simulink model "sampleModel63"  (R2021b)
settings: Solver=VariableStepAuto  StartTime=0.0  StopTime=10.0  RelTol=1e-3
undefined symbols (not defined in the file or in its folder): DiscIntNeverNeededParam, Newton, Raphson
libraries: simulink x12, slpidlib x2
settings Model: Creator=user  LastModifiedBy=user

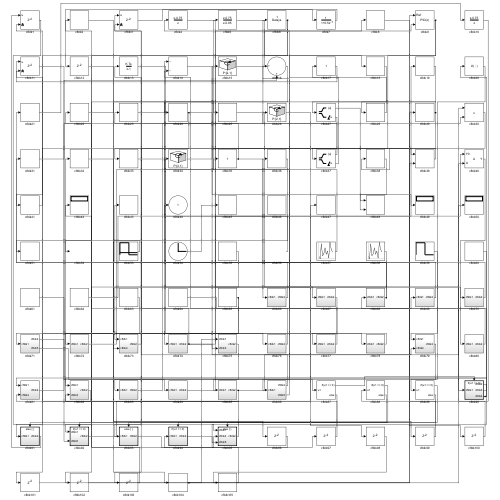
[thumbnail: Simulink's stored preview of the top-level diagram]
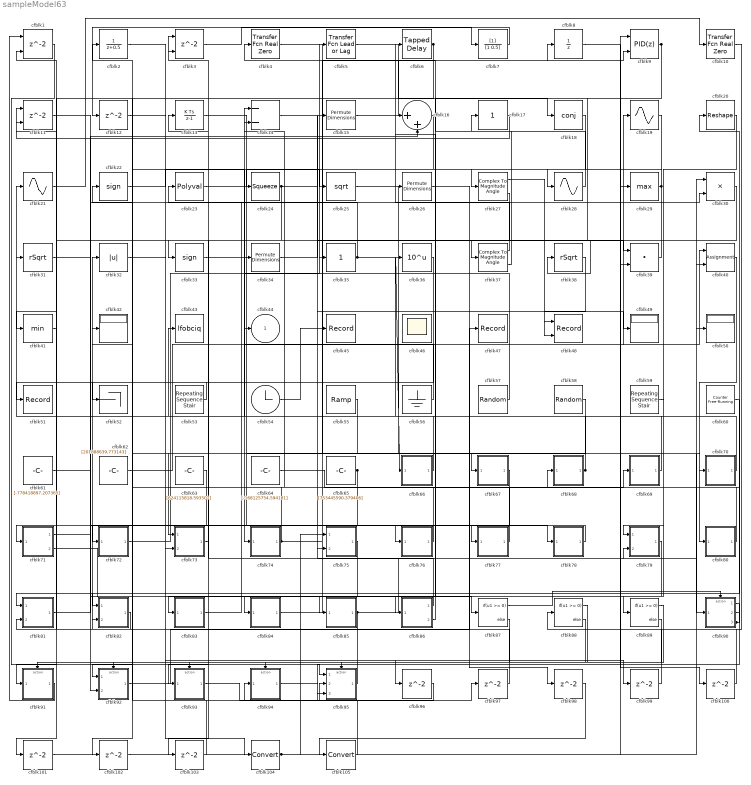
== system sampleModel63 ==
  cfblk1 : Delay  ShowEnablePort=on  SampleTime=1
      settings: InputPortMap=u0,e6
  cfblk10 : simulink/Discrete/Transfer Fcn Real Zero  ZeroZ=0.75  ICPrevInput=0.0  DoSatur=off
      settings: SourceProductBaseCode=SL
  cfblk{12,96..103} (9 alike) : Delay  SampleTime=1
  cfblk104 : DataTypeConversion
  cfblk105 : DataTypeConversion
  cfblk11 : Delay  ShowEnablePort=on  SampleTime=1
      settings: InputPortMap=u0,e6
  cfblk13 : DiscreteIntegrator  ICPrevOutput=DiscIntNeverNeededParam  ICPrevScaledInput=DiscIntNeverNeededParam
  cfblk14 : Sum  Inputs=--
  cfblk15 : PermuteDimensions
  cfblk16 : Sum  Inputs=|++
  cfblk17 : simulink/Math Operations/Slider Gain  gain=1  low=0  high=2
  cfblk18 : Math  Operator=conj  SaturateOnIntegerOverflow=on
  cfblk19 : Sin  TimeSource=Use external signal  SampleTime=0
  cfblk2 : DiscreteTransferFcn  SampleTime=1
  cfblk20 : Reshape
  cfblk21 : Sin  TimeSource=Use external signal  SampleTime=0
  cfblk22 : Signum
  cfblk23 : Polyval  Coefs=[ +2.081618890e-019, -1.441693666e-014, +4.719686976e-010, -8.536869453e-006, +1.621573104e-001, -8.087801117e+001 ]
  cfblk24 : Squeeze
  cfblk25 : Sqrt  SaturateOnIntegerOverflow=on
  cfblk26 : PermuteDimensions
  cfblk27 : ComplexToMagnitudeAngle
  cfblk28 : Sin  TimeSource=Use external signal  SampleTime=0
  cfblk29 : MinMax  Function=max
  cfblk3 : Delay  ShowEnablePort=on  SampleTime=1
      settings: InputPortMap=u0,e6
  cfblk30 : Product  Inputs=**
  cfblk31 : Sqrt  Operator=rSqrt  AlgorithmType=Newton-Raphson  SaturateOnIntegerOverflow=on
  cfblk32 : Abs
  cfblk33 : Signum
  cfblk34 : PermuteDimensions
  cfblk35 : simulink/Math Operations/Slider Gain  gain=1  low=0  high=2
  cfblk36 : Math  Operator=10^u  SaturateOnIntegerOverflow=on
  cfblk37 : ComplexToMagnitudeAngle
  cfblk38 : Sqrt  Operator=rSqrt  AlgorithmType=Newton-Raphson  SaturateOnIntegerOverflow=on
  cfblk39 : DotProduct  InputSameDT=on  OutDataTypeStr=Inherit: Inherit via internal rule
  cfblk4 : simulink/Discrete/Transfer Fcn Real Zero  ZeroZ=0.75  ICPrevInput=0.0  DoSatur=off
      settings: SourceProductBaseCode=SL
  cfblk40 : Assignment  DiagnosticForDimensions=Warning  IndexOptions=Index vector (dialog)  Indices=1  OutputSizes=1
  cfblk41 : MinMax
  cfblk42 : Display
  cfblk43 : ToWorkspace  VariableName=lfobciq  SaveFormat=Timeseries  SampleTime=-1
  cfblk45 : Record  FileSettingsInternal="{\"entries\":[{\"content\":{\"excelSettings\":{\"content\":{},\"type\":\"Streamout.ExcelSettings\"}},\"type\":\"Streamout.FileSettingStorage\",\"uuid\":\"eab00038-920a-4507-b0a5-0f8dc5558c4e\"}],\"packageUris\":[\"http://schema.mathworks.com/mf0/streamout_blocks/R2020a\"],\"version\":\"1.0\"}"  SignalsInternal="{\"entries\":[{\"content\":{\"signals\":[{\"content\":{\"blockPath\":[\"sampleModel63/cfblk45\"],\"channel\":[],\"dimensions\":[1],\"domain\":\"sampleModel63/cfblk45\",\"lineColor\":\"#7e2f8e\",\"plots\":[1],\"port\":1,\"sid\":[\"\"],\"signalID\":2453,\"signalName\":\"cfblk54\"},\"type\":\"RecordBlkView.Signal\",\"uuid\":\"6f20d37a-a5dd-4b7e-9677-872bf411aa66\"}]},\"type\":\"RecordBlkView.InputSignals\",\"uuid\":\"9bafe70f-6cc7-4dfb-b2fd-3a91eeb87f2c\"}],\"packageUris\":[\"http://schema.mathworks.com/mf0/streamout_blocks/R2020a\"],\"version\":\"1.0\"}"  VisualizationBindings="{\"sparklinesplugin\":{\"info\":[{\"bindingParametersList\":[],\"subplotID\":1}]}}"
  cfblk46 : Scope
      settings: Floating=on
  cfblk47 : Record  FileSettingsInternal="{\"entries\":[{\"content\":{\"excelSettings\":{\"content\":{},\"type\":\"Streamout.ExcelSettings\"}},\"type\":\"Streamout.FileSettingStorage\",\"uuid\":\"8624b493-b75b-4048-a20b-65c7ffb17f01\"}],\"packageUris\":[\"http://schema.mathworks.com/mf0/streamout_blocks/R2020a\"],\"version\":\"1.0\"}"  SignalsInternal="{\"entries\":[{\"content\":{\"signals\":[{\"content\":{\"blockPath\":[\"sampleModel63/cfblk47\"],\"channel\":[],\"dimensions\":[1],\"domain\":\"sampleModel63/cfblk47\",\"lineColor\":\"#0072bd\",\"plots\":[1],\"port\":1,\"sid\":[\"\"],\"signalID\":2441,\"signalName\":\"cfblk92\"},\"type\":\"RecordBlkView.Signal\",\"uuid\":\"a7be9c3a-7afb-4874-9450-2f20fa88f380\"}]},\"type\":\"RecordBlkView.InputSignals\",\"uuid\":\"be4317a2-c2d3-43f3-bc84-726c03d485cb\"}],\"packageUris\":[\"http://schema.mathworks.com/mf0/streamout_blocks/R2020a\"],\"version\":\"1.0\"}"  VisualizationBindings="{\"sparklinesplugin\":{\"info\":[{\"bindingParametersList\":[],\"subplotID\":1}]}}"
  cfblk48 : Record  FileSettingsInternal="{\"entries\":[{\"content\":{\"excelSettings\":{\"content\":{},\"type\":\"Streamout.ExcelSettings\"}},\"type\":\"Streamout.FileSettingStorage\",\"uuid\":\"a40df8e6-25e3-4f39-8082-43196c5c9d58\"}],\"packageUris\":[\"http://schema.mathworks.com/mf0/streamout_blocks/R2020a\"],\"version\":\"1.0\"}"  Layout=[1 1]  SignalsInternal="{\"entries\":[{\"content\":{\"signals\":[{\"content\":{\"blockPath\":[\"sampleModel63/cfblk48\"],\"channel\":[],\"dimensions\":[1,1],\"domain\":\"sampleModel63/cfblk48\",\"lineColor\":\"#a2142f\",\"plots\":[1],\"port\":1,\"sid\":[\"\"],\"signalID\":2445,\"signalName\":\"cfblk27:1\"},\"type\":\"RecordBlkView.Signal\",\"uuid\":\"b3ce3bcc-e12a-4239-8f85-80006c98ae86\"},{\"content\":{\"blockPath\":[\"sampleModel63/cfblk48\"],\"channel\":[],\"dimensions\":[1,1],\"domain\":\"sampleModel63/cfblk48\",\"lineColor\":\"#139fff\",\"plots\":[1],\"port\":2,\"sid\":[\"\"],\"signalID\":2449,\"signalName\":\"cfblk38\"},\"type\":\"RecordBlkView.Signal\",\"uuid\":\"d8960520-a3b1-4adb-9b58-2e04172c18e8\"}]},\"type\":\"RecordBlkView.InputSignals\",\"uuid\":\"834f0da8-eec6-4e4f-9565-3c19297e5a2d\"}],\"packageUris\":[\"http://schema.mathworks.com/mf0/streamout_blocks/R2020a\"],\"version\":\"1.0\"}"  VisualizationBindings="{\"xyplotplugin\":{\"info\":[{\"series\":[{\"bindingParametersList\":[{\"parameter\":\"X-Axis\",\"signalID\":2445,\"signalName\":\"cfblk27:1\"},{\"parameter\":\"Y-Axis\",\"signalID\":2449,\"signalName\":\"cfblk38\"}],\"seriesID\":5141}],\"subplotID\":1}]}}"  CompatibilityTag=XY
  cfblk49 : Display
  cfblk5 : simulink/Discrete/Transfer Fcn Lead or Lag  PoleZ=0.95  ZeroZ=0.75  ICPrevOutput=0.0  ICPrevInput=0.0  DoSatur=off
      settings: SourceProductBaseCode=SL
  cfblk50 : Display
  cfblk51 : Record  FileSettingsInternal="{\"entries\":[{\"content\":{\"excelSettings\":{\"content\":{},\"type\":\"Streamout.ExcelSettings\"}},\"type\":\"Streamout.FileSettingStorage\",\"uuid\":\"85545bd8-52c1-4d99-9c40-672c6dfcf42a\"}],\"packageUris\":[\"http://schema.mathworks.com/mf0/streamout_blocks/R2020a\"],\"version\":\"1.0\"}"  SignalsInternal="{\"entries\":[{\"content\":{\"signals\":[{\"content\":{\"blockPath\":[\"sampleModel63/cfblk51\"],\"channel\":[],\"dimensions\":[1],\"domain\":\"sampleModel63/cfblk51\",\"lineColor\":\"#77ac30\",\"plots\":[1],\"port\":1,\"sid\":[\"\"],\"signalID\":2457,\"signalName\":\"cfblk53\"},\"type\":\"RecordBlkView.Signal\",\"uuid\":\"2fbab494-daff-4625-9a56-065129460eaf\"}]},\"type\":\"RecordBlkView.InputSignals\",\"uuid\":\"dac925e5-03f2-4dde-8f24-8a4a20c8e071\"}],\"packageUris\":[\"http://schema.mathworks.com/mf0/streamout_blocks/R2020a\"],\"version\":\"1.0\"}"  VisualizationBindings="{\"sparklinesplugin\":{\"info\":[{\"bindingParametersList\":[],\"subplotID\":1}]}}"
  cfblk52 : Terminator
  cfblk53 : simulink/Sources/Repeating Sequence Stair  OutValues=[503450450.521379, -107905093.515396]  tsamp=-1  OutMin=[]  OutMax=[]  OutDataTypeStr=double  OutputDataTypeScalingMode=double  OutDataType=fixdt(0,8)  ConRadixGroup=Best Precision: Vector-wise  OutScaling=2^-12
  cfblk54 : Clock
  cfblk55 : simulink/Sources/Ramp  slope=[-5371.335129]  start=[28.819203]  InitialOutput=[-574228.703144]
  cfblk56 : Ground
  cfblk57 : UniformRandomNumber  Minimum=[-7281642111.005922]  Maximum=[1759054305.272253]  Seed=[77560895.000000]  SampleTime=0.1
  cfblk58 : UniformRandomNumber  Minimum=[-9181369548.878405]  Maximum=[5487264494.618241]  Seed=[73205660.000000]  SampleTime=0.1
  cfblk59 : simulink/Sources/Repeating Sequence Stair  OutValues=[306494964.090970, 306068425.132044]  tsamp=-1  OutMin=[]  OutMax=[]  OutDataTypeStr=double  OutputDataTypeScalingMode=double  OutDataType=fixdt(0,8)  ConRadixGroup=Best Precision: Vector-wise  OutScaling=2^-12
  cfblk6 : simulink/Discrete/Tapped Delay  vinit=0.0  samptime=-1  NumDelays=1  DelayOrder=Oldest  includeCurrent=off
  cfblk60 : simulink/Sources/Counter Free-Running  NumBits=[41.000000]  tsamp=-1
  cfblk61 : Constant  Value=[-778418897.207365]  SampleTime=1
  cfblk62 : Constant  Value=[201888639.773143]  SampleTime=1
  cfblk63 : Constant  Value=[624115818.593507]  SampleTime=1
  cfblk64 : Constant  Value=[-168125754.594181]  SampleTime=1
  cfblk65 : Constant  Value=[753445590.379406]  SampleTime=1
  cfblk66 : Subsystem
  cfblk67 : Subsystem
  cfblk68 : Subsystem
  cfblk69 : Subsystem
  cfblk7 : DiscreteFilter  SampleTime=1
  cfblk70 : Subsystem
  cfblk71 : Subsystem
  cfblk72 : Subsystem
  cfblk73 : Subsystem
  cfblk74 : Subsystem
  cfblk75 : Subsystem
  cfblk76 : Subsystem
  cfblk77 : Subsystem
  cfblk78 : Subsystem
  cfblk79 : Subsystem
  cfblk8 : UnitDelay  HasFrameUpgradeWarning=on
  cfblk80 : Subsystem
  cfblk81 : Subsystem
  cfblk82 : Subsystem
  cfblk83 : Subsystem
  cfblk84 : Subsystem
  cfblk85 : Subsystem
  cfblk86 : Subsystem
  cfblk87 : If  IfExpression=u1 >= 0  SampleTime=1
  cfblk88 : If  IfExpression=u1 >= 0  SampleTime=1
  cfblk89 : If  IfExpression=u1 >= 0  SampleTime=1
  cfblk9 : slpidlib/PID Controller (2DOF)  Controller=PID  Form=Parallel  TimeDomain=Discrete-time  UseExternalTs=off  SampleTime=1  IntegratorMethod=Forward Euler  FilterMethod=Forward Euler  ControllerParametersSource=internal  P=1  I=1  D=0  UseFilter=on  N=100  b=1  c=1  TunerSelectOption=Transfer Function Based (PID Tuner App)  InitialConditionSource=internal  InitialConditionForIntegrator=0  InitialConditionForFilter=0  DifferentiatorICPrevScaledInput=0  ExternalReset=none  TrackingMode=off  Kt=1  LimitOutput=off  SatLimitsSource=internal  UpperSaturationLimit=inf  LowerSaturationLimit=-inf  LinearizeAsGain=off  AntiWindupMode=none  Kb=1  POutMin=[]  POutMax=[]  IOutMin=[]  IOutMax=[]  DOutMin=[]  DOutMax=[]  NOutMin=[]  NOutMax=[]  bOutMin=[]  bOutMax=[]  cOutMin=[]  cOutMax=[]  SumOutMin=[]  SumOutMax=[]  SaturationOutMin=[]  SaturationOutMax=[]  PParamMin=[]  PParamMax=[]  IParamMin=[]  IParamMax=[]  DParamMin=[]  DParamMax=[]  NParamMin=[]  NParamMax=[]  bParamMin=[]  bParamMax=[]  cParamMin=[]  cParamMax=[]  KbParamMin=[]  KbParamMax=[]  KtParamMin=[]  KtParamMax=[]  KbOutMin=[]  KbOutMax=[]  KtOutMin=[]  KtOutMax=[]  IntegratorOutMin=[]  IntegratorOutMax=[]  FilterOutMin=[]  FilterOutMax=[]  SumI1OutMin=[]  SumI1OutMax=[]  SumI2OutMin=[]  SumI2OutMax=[]  SumI3OutMin=[]  SumI3OutMax=[]  SumI4OutMin=[]  SumI4OutMax=[]  SumDOutMin=[]  SumDOutMax=[]  Sum1OutMin=[]  Sum1OutMax=[]  Sum2OutMin=[]  Sum2OutMax=[]  Sum3OutMin=[]  Sum3OutMax=[]  DifferentiatorOutMin=[]  DifferentiatorOutMax=[]  FilterDiffOutCoefMin=[]  FilterDiffOutCoefMax=[]  ReciprocalOutMin=[]  ReciprocalOutMax=[]  SumDenOutMin=[]  SumDenOutMax=[]  SumNumOutMin=[]  SumNumOutMax=[]  DivideOutMin=[]  DivideOutMax=[]  UdiffTsProdOutMin=[]  UdiffTsProdOutMax=[]  NTsProdOutMin=[]  NTsProdOutMax=[]  UintegralTsProdOutMin=[]  UintegralTsProdOutMax=[]  UngainTsProdOutMin=[]  UngainTsProdOutMax=[]  IntegratorContinuousStateAttributes=''  IntegratorStateMustResolveToSignalObject=off  IntegratorRTWStateStorageClass=Auto  FilterContinuousStateAttributes=''  FilterStateMustResolveToSignalObject=off  FilterRTWStateStorageClass=Auto  ParallelPVariant=InternalParameters  IdealPVariant=Disabled  IVariant=InternalParameters  DVariant=InternalParameters  bVariant=InternalParameters  cVariant=InternalParameters  IntegratorVariant=Discrete  SatVariant=Disabled  AWVariant=Passthrough  PCopyVariant=Disabled  TRVariant=Disabled  FdbkBlocksVariant=Forward  IdealPFdbkVariant=Disabled  SatFdbkVariant=Disabled  DerivativeFilterVariant=ForwardEulerFilter  NVariant=InternalParameters  NCopyVariant=Disabled  FilterICVariant=InternalICsFilter  IntegratorICVariant=InternalICs  ExternalResetVariant=Disabled  TRSumVariant=Passthrough  SumFdbkVariant=Disabled  SumVariant=Sum_PID  TsampFilterVariant=InternalTs  TsampNgainVariant=Passthrough  TsampIntegralVariant=Passthrough  ExternalSaturationOutDataTypeStr=Inherit: Same as second input
      settings: SourceProductBaseCode=SL
  cfblk90 : Subsystem  TreatAsAtomicUnit=on
  cfblk91 : Subsystem  TreatAsAtomicUnit=on
  cfblk92 : Subsystem  TreatAsAtomicUnit=on
  cfblk93 : Subsystem  TreatAsAtomicUnit=on
  cfblk94 : Subsystem  TreatAsAtomicUnit=on
  cfblk95 : Subsystem  TreatAsAtomicUnit=on
  cfblk44 : Outport
  wires:
  cfblk28/1 -> cfblk4/1
  cfblk40/1 -> cfblk80/1(cfblk1)
  cfblk24/1 -> cfblk49/1, cfblk103/1
  cfblk60/1 -> cfblk81/1(cfblk1)
  cfblk9/1 -> cfblk33/1, cfblk86/1(cfblk1)
  cfblk1/1 -> cfblk95/1(cfblk1)
  cfblk68/1(cfblk2) -> cfblk21/1, cfblk36/1
  cfblk35/1 -> cfblk66/1(cfblk1), cfblk3/2
  cfblk4/1 -> cfblk67/1(cfblk1)
  cfblk29/1 -> cfblk38/1, cfblk27/1
  cfblk82/1(cfblk2) -> cfblk81/2(cfblk4)
  cfblk25/1 -> cfblk90/1(cfblk1)
  cfblk10/1 -> cfblk88/1
  cfblk70/1(cfblk2) -> cfblk31/1
  cfblk7/1 -> cfblk12/1
  cfblk95/1(cfblk2) -> cfblk32/1
  cfblk27/1 -> cfblk48/1
  cfblk64/1 -> cfblk69/1(cfblk1)
  cfblk20/1 -> cfblk89/1
  cfblk72/1(cfblk2) -> cfblk5/1
  cfblk69/1(cfblk2) -> cfblk14/1
  cfblk3/1 -> cfblk7/1
  cfblk75/1(cfblk2) -> cfblk83/1(cfblk1)
  cfblk21/1 -> cfblk10/1
  cfblk84/1(cfblk2) -> cfblk9/2
  cfblk53/1 -> cfblk51/1
  cfblk18/1 -> cfblk74/1(cfblk1)
  cfblk54/1 -> cfblk45/1
  cfblk62/1 -> cfblk19/1
  cfblk30/1 -> cfblk41/1
  cfblk57/1 -> cfblk35/1
  cfblk11/1 -> cfblk78/1(cfblk1)
  cfblk5/1 -> cfblk18/1
  cfblk78/1(cfblk2) -> cfblk71/1(cfblk1)
  cfblk34/1 -> cfblk15/1
  cfblk19/1 -> cfblk28/1
  cfblk65/1 -> cfblk72/1(cfblk1), cfblk93/1(cfblk1)
  cfblk92/1(cfblk2) -> cfblk47/1
  cfblk73/1(cfblk2) -> cfblk3/1
  cfblk67/1(cfblk2) -> cfblk77/1(cfblk1)
  cfblk93/1(cfblk2) -> cfblk95/2(cfblk4)
  cfblk13/1 -> cfblk76/1(cfblk1)
  cfblk14/1 -> cfblk39/1
  cfblk63/1 -> cfblk91/1(cfblk1)
  cfblk90/1(cfblk2) -> cfblk95/3(cfblk5)
  cfblk6/1 -> cfblk101/1, cfblk102/1
  cfblk16/1 -> cfblk52/1
  cfblk74/1(cfblk2) -> cfblk40/1, cfblk42/1, cfblk79/2(cfblk4)
  cfblk71/1(cfblk2) -> cfblk84/1(cfblk1)
  cfblk37/1 -> cfblk6/1
  cfblk79/1(cfblk2) -> cfblk85/1(cfblk1)
  cfblk66/1(cfblk2) -> cfblk43/1
  cfblk33/1 -> cfblk70/1(cfblk1)
  cfblk37/2 -> cfblk17/1
  cfblk55/1 -> cfblk73/1(cfblk1)
  cfblk41/1 -> cfblk11/1
  cfblk71/2(cfblk5) -> cfblk87/1
  cfblk36/1 -> cfblk73/2(cfblk4)
  cfblk15/1 -> cfblk8/1
  cfblk39/1 -> cfblk37/1
  cfblk2/1 -> cfblk104/1
  cfblk56/1 -> cfblk44/1
  cfblk91/1(cfblk2) -> cfblk1/1
  cfblk77/1(cfblk2) -> cfblk16/1
  cfblk27/2 -> cfblk75/2(cfblk3)
  cfblk90/2(cfblk3) -> cfblk82/1(cfblk1)
  cfblk86/1(cfblk2) -> cfblk23/1
  cfblk23/1 -> cfblk25/1
  cfblk90/3(cfblk4) -> cfblk68/1(cfblk1), cfblk20/1
  cfblk59/1 -> cfblk79/1(cfblk1)
  cfblk76/1(cfblk2) -> cfblk14/2
  cfblk22/1 -> cfblk24/1
  cfblk31/1 -> cfblk16/2
  cfblk81/1(cfblk2) -> cfblk26/1
  cfblk85/1(cfblk2) -> cfblk50/1, cfblk82/2(cfblk3)
  cfblk17/1 -> cfblk11/2
  cfblk80/1(cfblk2) -> cfblk13/1
  cfblk83/1(cfblk2) -> cfblk30/2
  cfblk58/1 -> cfblk92/1(cfblk1)
  cfblk38/1 -> cfblk48/2
  cfblk86/2(cfblk5) -> cfblk34/1
  cfblk61/1 -> cfblk92/2(cfblk5)
  cfblk87/1 -> cfblk90/Action
  cfblk87/2 -> cfblk91/Action
  cfblk88/1 -> cfblk92/Action
  cfblk88/2 -> cfblk93/Action
  cfblk89/1 -> cfblk94/Action
  cfblk89/2 -> cfblk95/Action
  cfblk32/1 -> cfblk96/1
  cfblk96/1 -> cfblk94/1(cfblk1)
  cfblk94/1(cfblk2) -> cfblk97/1
  cfblk97/1 -> cfblk1/2
  cfblk26/1 -> cfblk98/1
  cfblk12/1 -> cfblk99/1
  cfblk99/1 -> cfblk9/1
  cfblk8/1 -> cfblk100/1
  cfblk100/1 -> cfblk30/1
  cfblk101/1 -> cfblk39/2
  cfblk102/1 -> cfblk40/2
  cfblk103/1 -> cfblk22/1
  cfblk104/1 -> cfblk29/1, cfblk75/1(cfblk1)
  cfblk98/1 -> cfblk105/1
  cfblk105/1 -> cfblk2/1

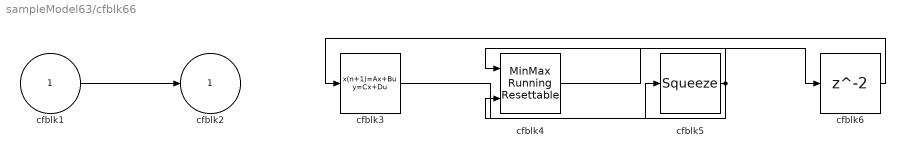
== system sampleModel63/cfblk66 ==
  cfblk1 : Inport
  cfblk3 : DiscreteStateSpace
  cfblk4 : simulink/Math Operations/MinMax Running Resettable  Function=min  vinit=0.0
  cfblk5 : Squeeze
  cfblk6 : Delay  SampleTime=1
  cfblk2 : Outport
  wires:
  cfblk5/1 -> cfblk4/1, cfblk4/2
  cfblk3/1 -> cfblk5/1
  cfblk1/1 -> cfblk2/1
  cfblk4/1 -> cfblk6/1
  cfblk6/1 -> cfblk3/1

== system sampleModel63/cfblk67 ==
  cfblk1 : Inport
  cfblk3 : DiscreteStateSpace
  cfblk2 : Outport
  wires:
  cfblk1/1 -> cfblk2/1, cfblk3/1

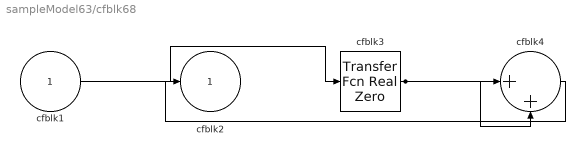
== system sampleModel63/cfblk68 ==
  cfblk1 : Inport
  cfblk3 : simulink/Discrete/Transfer Fcn Real Zero  ZeroZ=0.75  ICPrevInput=0.0  DoSatur=off
      settings: SourceProductBaseCode=SL
  cfblk4 : Sum  Inputs=|++
  cfblk2 : Outport
  wires:
  cfblk1/1 -> cfblk3/1
  cfblk4/1 -> cfblk2/1
  cfblk3/1 -> cfblk4/1, cfblk4/2

== system sampleModel63/cfblk69 ==
  cfblk1 : Inport
  cfblk3 : Sum  Inputs=+
  cfblk2 : Outport
  wires:
  cfblk1/1 -> cfblk3/1
  cfblk3/1 -> cfblk2/1

== system sampleModel63/cfblk70 ==
  cfblk1 : Inport
  cfblk3 : Constant  Value=[-469979118.502152]  SampleTime=1
  cfblk2 : Outport
  wires:
  cfblk1/1 -> cfblk2/1

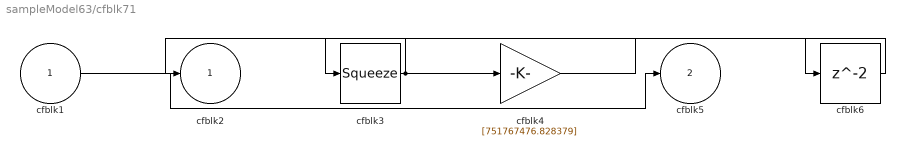
== system sampleModel63/cfblk71 ==
  cfblk1 : Inport
  cfblk3 : Squeeze
  cfblk4 : Gain  Gain=[751767476.828379]
  cfblk6 : Delay  SampleTime=1
  cfblk2 : Outport
  cfblk5 : Outport  Port=2
  wires:
  cfblk1/1 -> cfblk5/1
  cfblk3/1 -> cfblk2/1, cfblk4/1
  cfblk4/1 -> cfblk6/1
  cfblk6/1 -> cfblk3/1

== system sampleModel63/cfblk72 ==
  cfblk1 : Inport
  cfblk3 : Sin  TimeSource=Use external signal  SampleTime=0
  cfblk2 : Outport
  wires:
  cfblk1/1 -> cfblk3/1
  cfblk3/1 -> cfblk2/1

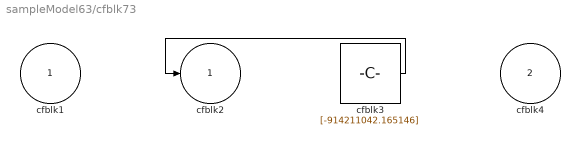
== system sampleModel63/cfblk73 ==
  cfblk1 : Inport
  cfblk4 : Inport  Port=2
  cfblk3 : Constant  Value=[-914211042.165146]  SampleTime=1
  cfblk2 : Outport
  wires:
  cfblk3/1 -> cfblk2/1

== system sampleModel63/cfblk74 ==
  cfblk1 : Inport
  cfblk3 : Bias  Bias=[-714518789.480261]
  cfblk2 : Outport
  wires:
  cfblk3/1 -> cfblk2/1
  cfblk1/1 -> cfblk3/1

== system sampleModel63/cfblk75 ==
  cfblk1 : Inport
  cfblk3 : Inport  Port=2
  cfblk2 : Outport
  wires:
  cfblk3/1 -> cfblk2/1

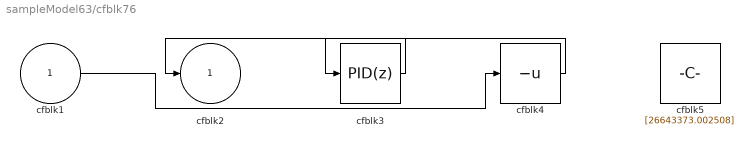
== system sampleModel63/cfblk76 ==
  cfblk1 : Inport
  cfblk3 : slpidlib/PID Controller  Controller=PID  Form=Parallel  TimeDomain=Discrete-time  UseExternalTs=off  SampleTime=1  IntegratorMethod=Forward Euler  FilterMethod=Forward Euler  ControllerParametersSource=internal  P=1  I=1  D=0  UseFilter=on  N=100  TunerSelectOption=Transfer Function Based (PID Tuner App)  InitialConditionSource=internal  InitialConditionForIntegrator=0  InitialConditionForFilter=0  DifferentiatorICPrevScaledInput=0  ExternalReset=none  TrackingMode=off  Kt=1  LimitOutput=off  SatLimitsSource=internal  UpperSaturationLimit=inf  LowerSaturationLimit=-inf  LinearizeAsGain=off  AntiWindupMode=none  Kb=1  POutMin=[]  POutMax=[]  IOutMin=[]  IOutMax=[]  DOutMin=[]  DOutMax=[]  NOutMin=[]  NOutMax=[]  SumOutMin=[]  SumOutMax=[]  SaturationOutMin=[]  SaturationOutMax=[]  PParamMin=[]  PParamMax=[]  IParamMin=[]  IParamMax=[]  DParamMin=[]  DParamMax=[]  NParamMin=[]  NParamMax=[]  KbParamMin=[]  KbParamMax=[]  KtParamMin=[]  KtParamMax=[]  KbOutMin=[]  KbOutMax=[]  KtOutMin=[]  KtOutMax=[]  IntegratorOutMin=[]  IntegratorOutMax=[]  FilterOutMin=[]  FilterOutMax=[]  SumI1OutMin=[]  SumI1OutMax=[]  SumI2OutMin=[]  SumI2OutMax=[]  SumI3OutMin=[]  SumI3OutMax=[]  SumI4OutMin=[]  SumI4OutMax=[]  SumDOutMin=[]  SumDOutMax=[]  DifferentiatorOutMin=[]  DifferentiatorOutMax=[]  FilterDiffOutCoefMin=[]  FilterDiffOutCoefMax=[]  ReciprocalOutMin=[]  ReciprocalOutMax=[]  SumDenOutMin=[]  SumDenOutMax=[]  SumNumOutMin=[]  SumNumOutMax=[]  DivideOutMin=[]  DivideOutMax=[]  UdiffTsProdOutMin=[]  UdiffTsProdOutMax=[]  NTsProdOutMin=[]  NTsProdOutMax=[]  UintegralTsProdOutMin=[]  UintegralTsProdOutMax=[]  UngainTsProdOutMin=[]  UngainTsProdOutMax=[]  IntegratorContinuousStateAttributes=''  IntegratorStateMustResolveToSignalObject=off  IntegratorRTWStateStorageClass=Auto  FilterContinuousStateAttributes=''  FilterStateMustResolveToSignalObject=off  FilterRTWStateStorageClass=Auto  ParallelPVariant=InternalParameters  IdealPVariant=Disabled  IVariant=InternalParameters  DVariant=InternalParameters  IntegratorVariant=Discrete  SatVariant=Disabled  AWVariant=Passthrough  PCopyVariant=Disabled  TRVariant=Disabled  FdbkBlocksVariant=Forward  IdealPFdbkVariant=Disabled  SatFdbkVariant=Disabled  DerivativeFilterVariant=ForwardEulerFilter  NVariant=InternalParameters  NCopyVariant=Disabled  FilterICVariant=InternalICsFilter  IntegratorICVariant=InternalICs  ExternalResetVariant=Disabled  TRSumVariant=Passthrough  SumFdbkVariant=Disabled  SumVariant=Sum_PID  TsampFilterVariant=InternalTs  TsampNgainVariant=Passthrough  TsampIntegralVariant=Passthrough  ExternalSaturationOutDataTypeStr=Inherit: Same as second input
  cfblk4 : UnaryMinus
  cfblk5 : Constant  Value=[26643373.002508]  SampleTime=1
  cfblk2 : Outport
  wires:
  cfblk3/1 -> cfblk2/1
  cfblk1/1 -> cfblk4/1
  cfblk4/1 -> cfblk3/1

== system sampleModel63/cfblk77 ==
  cfblk1 : Inport
  cfblk3 : DiscreteIntegrator  ICPrevOutput=DiscIntNeverNeededParam  ICPrevScaledInput=DiscIntNeverNeededParam
  cfblk4 : Constant  Value=[-108816634.393486]  SampleTime=1
  cfblk2 : Outport
  wires:
  cfblk1/1 -> cfblk2/1
  cfblk4/1 -> cfblk3/1

== system sampleModel63/cfblk78 ==
  cfblk1 : Inport
  cfblk3 : Constant  Value=[613475250.594673]  SampleTime=1
  cfblk2 : Outport
  wires:
  cfblk1/1 -> cfblk2/1

== system sampleModel63/cfblk79 ==
  cfblk1 : Inport
  cfblk4 : Inport  Port=2
  cfblk3 : Delay  DelayLengthSource=Input port  SampleTime=1
      settings: InputPortMap=u0,p1
  cfblk2 : Outport
  wires:
  cfblk1/1 -> cfblk3/1
  cfblk4/1 -> cfblk3/2
  cfblk3/1 -> cfblk2/1

== system sampleModel63/cfblk80 ==
  cfblk1 : Inport
  cfblk3 : DiscreteFilter  SampleTime=1
  cfblk2 : Outport
  wires:
  cfblk1/1 -> cfblk3/1
  cfblk3/1 -> cfblk2/1

== system sampleModel63/cfblk81 ==
  cfblk1 : Inport
  cfblk4 : Inport  Port=2
  cfblk3 : Math  Operator=transpose  SaturateOnIntegerOverflow=on
  cfblk2 : Outport
  wires:
  cfblk1/1 -> cfblk2/1
  cfblk4/1 -> cfblk3/1

== system sampleModel63/cfblk82 ==
  cfblk1 : Inport
  cfblk3 : Inport  Port=2
  cfblk2 : Outport
  wires:
  cfblk3/1 -> cfblk2/1

== system sampleModel63/cfblk83 ==
  cfblk1 : Inport
  cfblk3 : Math  Operator=log  SaturateOnIntegerOverflow=on
  cfblk2 : Outport
  wires:
  cfblk1/1 -> cfblk2/1, cfblk3/1

== system sampleModel63/cfblk84 ==
  cfblk1 : Inport
  cfblk3 : DiscreteFir  SampleTime=1
  cfblk2 : Outport
  wires:
  cfblk1/1 -> cfblk2/1, cfblk3/1

== system sampleModel63/cfblk85 ==
  cfblk1 : Inport
  cfblk3 : Bias  Bias=[-692510062.246402]
  cfblk2 : Outport
  wires:
  cfblk1/1 -> cfblk2/1, cfblk3/1

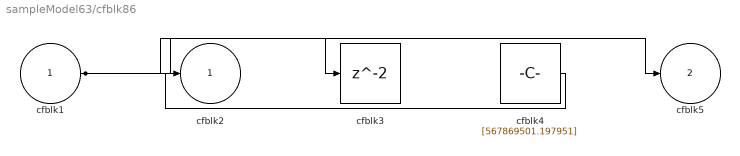
== system sampleModel63/cfblk86 ==
  cfblk1 : Inport
  cfblk3 : Delay  SampleTime=1
  cfblk4 : Constant  Value=[567869501.197951]  SampleTime=1
  cfblk2 : Outport
  cfblk5 : Outport  Port=2
  wires:
  cfblk1/1 -> cfblk5/1, cfblk3/1
  cfblk4/1 -> cfblk2/1

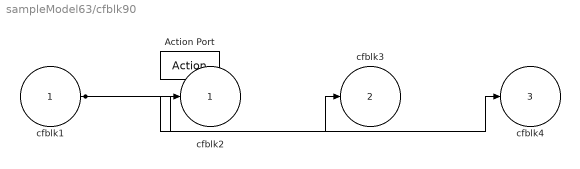
== system sampleModel63/cfblk90 ==
  cfblk1 : Inport
  Action Port : ActionPort  ActionPortLabel=if(u1 >= 0)
  cfblk2 : Outport
  cfblk3 : Outport  Port=2
  cfblk4 : Outport  Port=3
  wires:
  cfblk1/1 -> cfblk3/1, cfblk2/1, cfblk4/1

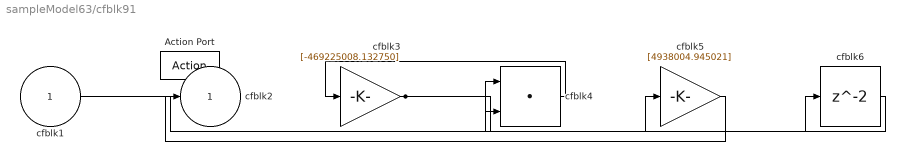
== system sampleModel63/cfblk91 ==
  cfblk1 : Inport
  Action Port : ActionPort  ActionPortLabel=else
  cfblk3 : Gain  Gain=[-469225008.132750]
  cfblk4 : DotProduct  InputSameDT=on  OutDataTypeStr=Inherit: Inherit via internal rule
  cfblk5 : Gain  Gain=[4938004.945021]
  cfblk6 : Delay
  cfblk2 : Outport
  wires:
  cfblk1/1 -> cfblk4/1
  cfblk5/1 -> cfblk2/1
  cfblk4/1 -> cfblk3/1
  cfblk3/1 -> cfblk5/1, cfblk6/1
  cfblk6/1 -> cfblk4/2

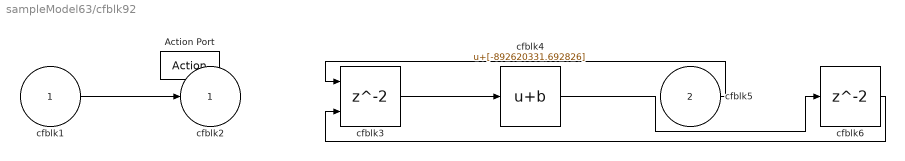
== system sampleModel63/cfblk92 ==
  cfblk1 : Inport
  cfblk5 : Inport  Port=2
  Action Port : ActionPort  ActionPortLabel=if(u1 >= 0)
  cfblk3 : Delay  ShowEnablePort=on
      settings: InputPortMap=u0,e6
  cfblk4 : Bias  Bias=[-892620331.692826]
  cfblk6 : Delay
  cfblk2 : Outport
  wires:
  cfblk1/1 -> cfblk2/1
  cfblk3/1 -> cfblk4/1
  cfblk5/1 -> cfblk3/1
  cfblk4/1 -> cfblk6/1
  cfblk6/1 -> cfblk3/2

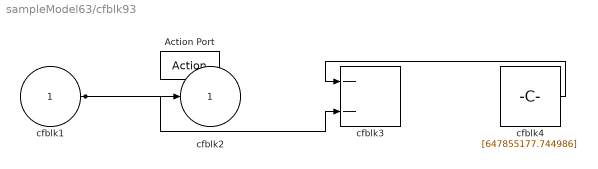
== system sampleModel63/cfblk93 ==
  cfblk1 : Inport
  Action Port : ActionPort  ActionPortLabel=else
  cfblk3 : Sum  Inputs=--
  cfblk4 : Constant  Value=[647855177.744986]  SampleTime=1
  cfblk2 : Outport
  wires:
  cfblk1/1 -> cfblk2/1, cfblk3/2
  cfblk4/1 -> cfblk3/1

== system sampleModel63/cfblk94 ==
  cfblk1 : Inport
  Action Port : ActionPort  ActionPortLabel=if(u1 >= 0)
  cfblk3 : Sum  Inputs=-+
  cfblk2 : Outport
  wires:
  cfblk1/1 -> cfblk3/1, cfblk3/2
  cfblk3/1 -> cfblk2/1

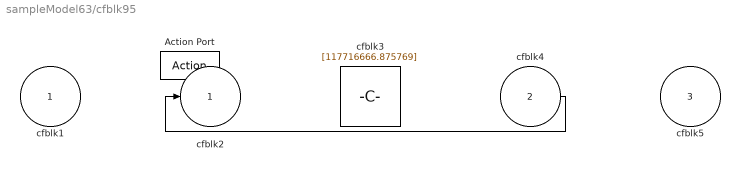
== system sampleModel63/cfblk95 ==
  cfblk1 : Inport
  cfblk4 : Inport  Port=2
  cfblk5 : Inport  Port=3
  Action Port : ActionPort  ActionPortLabel=else
  cfblk3 : Constant  Value=[117716666.875769]  SampleTime=1
  cfblk2 : Outport
  wires:
  cfblk4/1 -> cfblk2/1
